simulink model "Hw1P1b"  (R2017a)
settings: Solver=VariableStepAuto  StartTime=0.0  StopTime=10.0  RelTol=1e-3
settings Model: Creator=Soutrik  LastModifiedBy=Soutrik

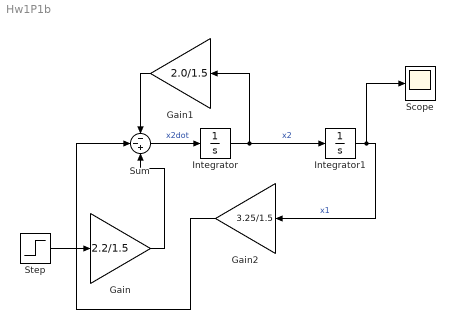
== system Hw1P1b ==
  Gain : Gain  Gain=2.2/1.5
  Gain1 : Gain  Gain=2.0/1.5
  Gain2 : Gain  Gain=3.25/1.5
  Integrator : Integrator
  Integrator1 : Integrator
  Scope : Scope
  Step : Step  SampleTime=0
  Sum : Sum  Inputs=--+
  wires:
  Integrator1/1 -> Scope/1, Gain2/1  "x1"
  Integrator/1 -> Gain1/1, Integrator1/1  "x2"
  Sum/1 -> Integrator/1  "x2dot"
  Step/1 -> Gain/1
  Gain/1 -> Sum/3
  Gain1/1 -> Sum/1
  Gain2/1 -> Sum/2
